simulink model "magnetic_levitation"  (R2015b)
settings: Solver=VariableStepAuto  StartTime=0.0  StopTime=1000  RelTol=1e-3
undefined symbols (not defined in the file or in its folder): magnetic_levitation_controller
settings Model: Creator=magiccjae  LastModifiedBy=magiccjae

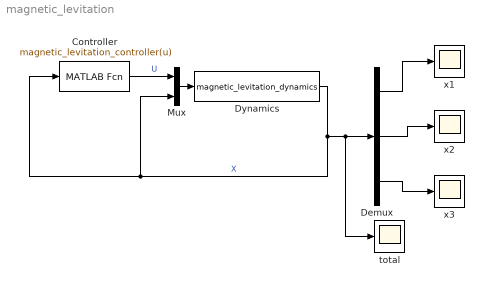
== system magnetic_levitation ==
  Controller : MATLABFcn  MATLABFcn=magnetic_levitation_controller(u)
  Demux : Demux  Outputs=3
  Dynamics : S-Function  FunctionName=magnetic_levitation_dynamics  SFunctionDeploymentMode=off  EnableBusSupport=off
  Mux : Mux  Inputs=[1 3]
  total : Scope
  x1 : Scope
  x2 : Scope
  x3 : Scope
  wires:
  Dynamics/1 -> total/1, Demux/1, Mux/2, Controller/1  "X"
  Controller/1 -> Mux/1  "U"
  Mux/1 -> Dynamics/1
  Demux/1 -> x1/1
  Demux/2 -> x2/1
  Demux/3 -> x3/1
